simulink model "WEC_Model_SIMU"  (R2023b)
settings: Solver=ode4  StartTime=0.0  StopTime=20  FixedStep=50e-6  RelTol=1e-3
InitFcn:
  | load('Pgridwec.mat')
  | Lg=0.05;
  | rg=0.01;
  | kp_g=0.5*10.9;
  | ki_g=0.1*7.9e4;
  | Sbase=100e6;
  | Imax=1.5;
  | Vbase=132e3;
  | Ibase=5248.639;
libraries: slpidlib x2, spsPLL3phLib x1, spsabctodq0Lib x1, spsdq0toabcLib x1
settings Model: Creator=podde  LastModifiedBy=barajale

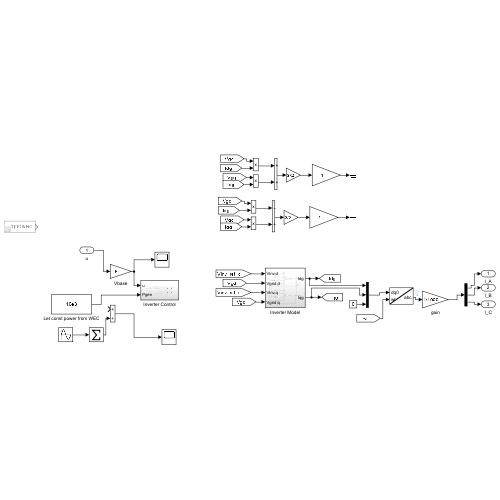
[thumbnail: Simulink's stored preview of the top-level diagram]
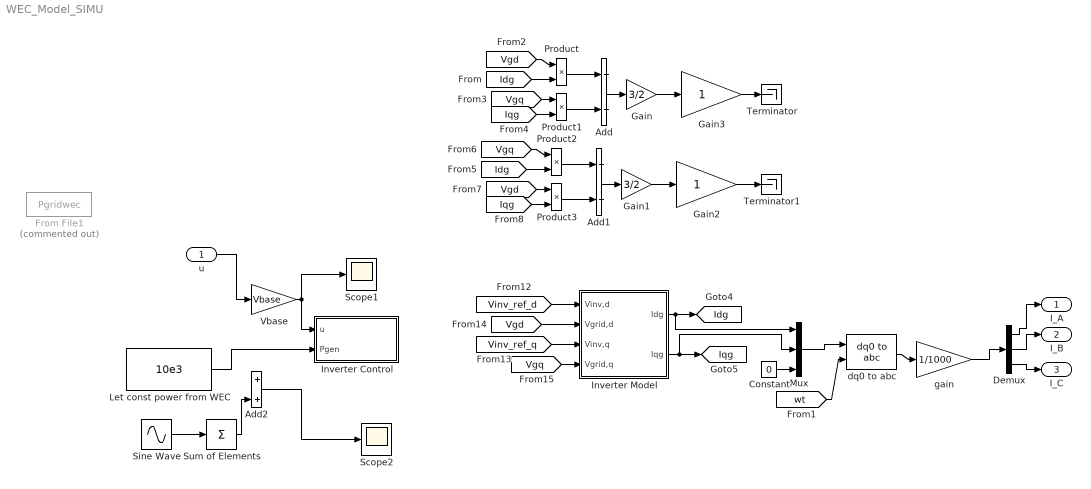
== system WEC_Model_SIMU ==
  u : Inport
  Add : Sum
  Add1 : Sum  Inputs=-+
  Add2 : Sum
  Constant : Constant  Value=0
  Demux : Demux  Outputs=3
  From File1 : FromFile  Commented=on  FileName=Pgridwec  SampleTime=0
  Gain : Gain  Gain=3/2
  Gain1 : Gain  Gain=3/2
  Gain2 : Gain
  Gain3 : Gain
  Inverter Control : Subsystem
  Inverter Model : Subsystem
  Let const power from WEC : Constant  Value=10e3
  Mux : Mux  Inputs=3
  Product{,1..3} (4 alike) : Product
  Scope1 : Scope
  Scope2 : Scope
  Sine Wave : Sin  Amplitude=0  Frequency=[2*pi/3 2*pi/5 2*pi/7]  Phase=[0,-2*pi/3, 2*pi/3]  SampleTime=0
  Sum of Elements : Sum  Inputs=+
  Terminator : Terminator
  Terminator1 : Terminator
  Vbase : Gain  Gain=Vbase
  dq0 to abc : spsdq0toabcLib/dq0 to abc  Alignment=90 degrees behind phase A axis
  gain : Gain  Gain=1/1000
  I_A : Outport
  I_B : Outport  Port=2
  I_C : Outport  Port=3
  tag scope: Idg=global, Iqg=global
  wires:
  Inverter Model/1(Idg) -> Mux/1, [Idg]
  Inverter Model/2(Iqg) -> Mux/2, [Iqg]
  [Vinv_ref_d] -> Inverter Model/1(Vinv,d)
  [Vgd] -> Inverter Model/2(Vgrid,d)
  [Vinv_ref_q] -> Inverter Model/3(Vinv,q)
  [Vgq] -> Inverter Model/4(Vgrid,q)
  Constant/1 -> Mux/3
  Mux/1 -> dq0 to abc/1
  [wt] -> dq0 to abc/2
  Demux/2 -> I_B/1
  Demux/3 -> I_C/1
  [Vgd] -> Product/1
  [Idg] -> Product/2
  [Vgq] -> Product1/1
  [Iqg] -> Product1/2
  Product/1 -> Add/1
  Product1/1 -> Add/2
  Add/1 -> Gain/1
  Product3/1 -> Add1/2
  [Vgq] -> Product2/1
  [Idg] -> Product2/2
  [Vgd] -> Product3/1
  Product2/1 -> Add1/1
  Add1/1 -> Gain1/1
  [Iqg] -> Product3/2
  Gain1/1 -> Gain2/1
  Gain2/1 -> Terminator1/1
  Gain/1 -> Gain3/1
  Gain3/1 -> Terminator/1
  Demux/1 -> I_A/1
  Vbase/1 -> Inverter Control/1(u), Scope1/1
  u/1 -> Vbase/1
  gain/1 -> Demux/1
  dq0 to abc/1 -> gain/1
  Sum of Elements/1 -> Add2/2
  Let const power from WEC/1 -> Inverter Control/2(Pgen)
  Add2/1 -> Scope2/1
  Sine Wave/1 -> Sum of Elements/1

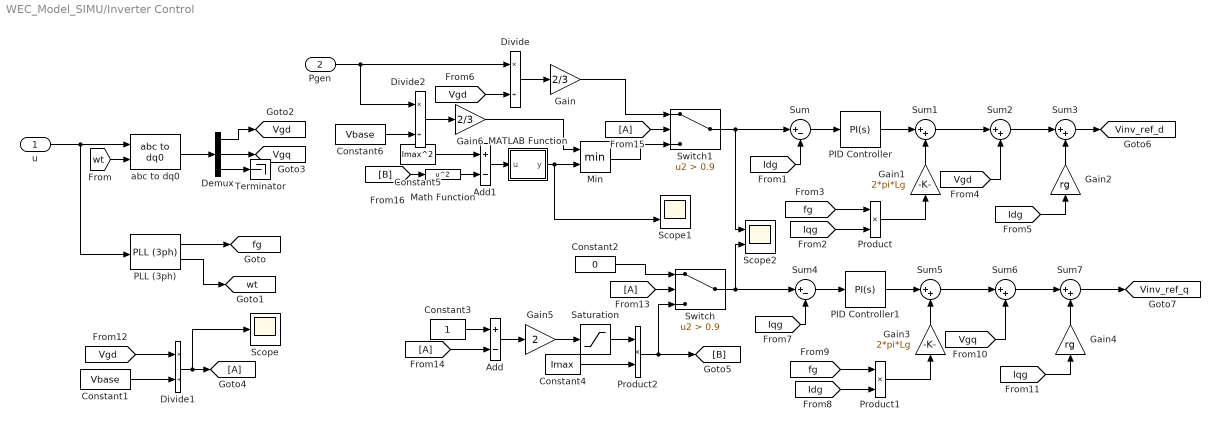
== system WEC_Model_SIMU/Inverter Control ==
  u : Inport
  Pgen : Inport  Port=2
  Add : Sum  Inputs=+-
  Add1 : Sum  Inputs=+-
  Constant1 : Constant  Value=Vbase
  Constant2 : Constant  Value=0
  Constant3 : Constant
  Constant4 : Constant  Value=Imax
  Constant5 : Constant  Value=Imax^2
  Constant6 : Constant  Value=Vbase
  Demux : Demux  Outputs=3
  Divide : Product  Inputs=*/
  Divide1 : Product  Inputs=*/
  Divide2 : Product  Inputs=*/
  From13 : From
  From14 : From
  From15 : From
  Gain : Gain  Gain=2/3
  Gain1 : Gain  Gain=2*pi*Lg
  Gain2 : Gain  Gain=rg
  Gain3 : Gain  Gain=2*pi*Lg
  Gain4 : Gain  Gain=rg
  Gain5 : Gain  Gain=2
  Gain6 : Gain  Gain=2/3
  Goto4 : Goto
  MATLAB Function : MATLAB Function  TreatAsAtomicUnit=on
  Math Function : Math  Operator=square
  Min : MinMax  Inputs=2
  PID Controller : slpidlib/PID Controller  Controller=PI  Form=Parallel  TimeDomain=Continuous-time  UseExternalTs=off  SampleTime=-1  IntegratorMethod=Forward Euler  FilterMethod=Forward Euler  ControllerParametersSource=internal  P=kp_g  I=ki_g  UseKiTs=off  D=0  N=100  UseFilter=on  TunerSelectOption=Transfer Function Based (PID Tuner App)  InitialConditionSource=internal  InitialConditionForIntegrator=0  InitialConditionForFilter=0  DifferentiatorICPrevScaledInput=0  ExternalReset=none  TrackingMode=off  Kt=1  LimitOutput=off  SatLimitsSource=internal  UpperSaturationLimit=inf  LowerSaturationLimit=-inf  LinearizeAsGain=on  AntiWindupMode=none  Kb=1  LimitIntegrator=off  UpperIntegratorSaturationLimit=inf  LowerIntegratorSaturationLimit=-inf  POutMin=[]  POutMax=[]  IOutMin=[]  IOutMax=[]  DOutMin=[]  DOutMax=[]  NOutMin=[]  NOutMax=[]  SumOutMin=[]  SumOutMax=[]  SaturationOutMin=[]  SaturationOutMax=[]  PParamMin=[]  PParamMax=[]  IParamMin=[]  IParamMax=[]  DParamMin=[]  DParamMax=[]  NParamMin=[]  NParamMax=[]  KbParamMin=[]  KbParamMax=[]  KtParamMin=[]  KtParamMax=[]  KbOutMin=[]  KbOutMax=[]  KtOutMin=[]  KtOutMax=[]  IntegratorOutMin=[]  IntegratorOutMax=[]  FilterOutMin=[]  FilterOutMax=[]  SumI1OutMin=[]  SumI1OutMax=[]  SumI2OutMin=[]  SumI2OutMax=[]  SumI3OutMin=[]  SumI3OutMax=[]  SumI4OutMin=[]  SumI4OutMax=[]  SumDOutMin=[]  SumDOutMax=[]  DifferentiatorOutMin=[]  DifferentiatorOutMax=[]  FilterDiffOutCoefMin=[]  FilterDiffOutCoefMax=[]  ReciprocalOutMin=[]  ReciprocalOutMax=[]  SumDenOutMin=[]  SumDenOutMax=[]  SumNumOutMin=[]  SumNumOutMax=[]  DivideOutMin=[]  DivideOutMax=[]  UdiffTsProdOutMin=[]  UdiffTsProdOutMax=[]  NTsProdOutMin=[]  NTsProdOutMax=[]  UintegralTsProdOutMin=[]  UintegralTsProdOutMax=[]  UngainTsProdOutMin=[]  UngainTsProdOutMax=[]  ClampingZeroOutDataTypeStr=Inherit: Inherit via back propagation  ClampingZeroOutMin=[]  ClampingZeroOutMax=[]  FilterDenConstantOutDataTypeStr=Inherit: Inherit via back propagation  FilterDenConstantOutMin=[]  FilterDenConstantOutMax=[]  PCopyOutDataTypeStr=Inherit: Inherit via back propagation  PCopyOutMin=[]  PCopyOutMax=[]  NCopyOutDataTypeStr=Inherit: Inherit via back propagation  NCopyOutMin=[]  NCopyOutMax=[]  IntegratorContinuousStateAttributes=''  IntegratorStateMustResolveToSignalObject=off  IntegratorRTWStateStorageClass=Auto  FilterContinuousStateAttributes=''  FilterStateMustResolveToSignalObject=off  FilterRTWStateStorageClass=Auto  ParallelPVariant=InternalParameters  IdealPVariant=Disabled  IVariant=InternalParameters  DVariant=Disabled  IntegratorVariant=Continuous  SatVariant=Disabled  AWVariant=Passthrough  PCopyVariant=Disabled  TRVariant=Disabled  FdbkBlocksVariant=Forward  IdealPFdbkVariant=Disabled  SatFdbkVariant=Disabled  DerivativeFilterVariant=Disabled  NVariant=Disabled  NCopyVariant=Disabled_SignalSpec  FilterICVariant=Disabled  IntegratorICVariant=InternalICs  ExternalResetVariant=Disabled  TRSumVariant=Passthrough  SumFdbkVariant=Disabled  SumVariant=Sum_PI  TsampFilterVariant=InternalTs  TsampNgainVariant=Passthrough  TsampIntegralVariant=Disabled_SignalSpec  ExternalSaturationOutDataTypeStr=Inherit: Same as second input
  PID Controller1 : slpidlib/PID Controller  Controller=PI  Form=Parallel  TimeDomain=Continuous-time  UseExternalTs=off  SampleTime=-1  IntegratorMethod=Forward Euler  FilterMethod=Forward Euler  ControllerParametersSource=internal  P=kp_g  I=ki_g  UseKiTs=off  D=0  N=100  UseFilter=on  TunerSelectOption=Transfer Function Based (PID Tuner App)  InitialConditionSource=internal  InitialConditionForIntegrator=0  InitialConditionForFilter=0  DifferentiatorICPrevScaledInput=0  ExternalReset=none  TrackingMode=off  Kt=1  LimitOutput=off  SatLimitsSource=internal  UpperSaturationLimit=inf  LowerSaturationLimit=-inf  LinearizeAsGain=on  AntiWindupMode=none  Kb=1  LimitIntegrator=off  UpperIntegratorSaturationLimit=inf  LowerIntegratorSaturationLimit=-inf  POutMin=[]  POutMax=[]  IOutMin=[]  IOutMax=[]  DOutMin=[]  DOutMax=[]  NOutMin=[]  NOutMax=[]  SumOutMin=[]  SumOutMax=[]  SaturationOutMin=[]  SaturationOutMax=[]  PParamMin=[]  PParamMax=[]  IParamMin=[]  IParamMax=[]  DParamMin=[]  DParamMax=[]  NParamMin=[]  NParamMax=[]  KbParamMin=[]  KbParamMax=[]  KtParamMin=[]  KtParamMax=[]  KbOutMin=[]  KbOutMax=[]  KtOutMin=[]  KtOutMax=[]  IntegratorOutMin=[]  IntegratorOutMax=[]  FilterOutMin=[]  FilterOutMax=[]  SumI1OutMin=[]  SumI1OutMax=[]  SumI2OutMin=[]  SumI2OutMax=[]  SumI3OutMin=[]  SumI3OutMax=[]  SumI4OutMin=[]  SumI4OutMax=[]  SumDOutMin=[]  SumDOutMax=[]  DifferentiatorOutMin=[]  DifferentiatorOutMax=[]  FilterDiffOutCoefMin=[]  FilterDiffOutCoefMax=[]  ReciprocalOutMin=[]  ReciprocalOutMax=[]  SumDenOutMin=[]  SumDenOutMax=[]  SumNumOutMin=[]  SumNumOutMax=[]  DivideOutMin=[]  DivideOutMax=[]  UdiffTsProdOutMin=[]  UdiffTsProdOutMax=[]  NTsProdOutMin=[]  NTsProdOutMax=[]  UintegralTsProdOutMin=[]  UintegralTsProdOutMax=[]  UngainTsProdOutMin=[]  UngainTsProdOutMax=[]  ClampingZeroOutDataTypeStr=Inherit: Inherit via back propagation  ClampingZeroOutMin=[]  ClampingZeroOutMax=[]  FilterDenConstantOutDataTypeStr=Inherit: Inherit via back propagation  FilterDenConstantOutMin=[]  FilterDenConstantOutMax=[]  PCopyOutDataTypeStr=Inherit: Inherit via back propagation  PCopyOutMin=[]  PCopyOutMax=[]  NCopyOutDataTypeStr=Inherit: Inherit via back propagation  NCopyOutMin=[]  NCopyOutMax=[]  IntegratorContinuousStateAttributes=''  IntegratorStateMustResolveToSignalObject=off  IntegratorRTWStateStorageClass=Auto  FilterContinuousStateAttributes=''  FilterStateMustResolveToSignalObject=off  FilterRTWStateStorageClass=Auto  ParallelPVariant=InternalParameters  IdealPVariant=Disabled  IVariant=InternalParameters  DVariant=Disabled  IntegratorVariant=Continuous  SatVariant=Disabled  AWVariant=Passthrough  PCopyVariant=Disabled  TRVariant=Disabled  FdbkBlocksVariant=Forward  IdealPFdbkVariant=Disabled  SatFdbkVariant=Disabled  DerivativeFilterVariant=Disabled  NVariant=Disabled  NCopyVariant=Disabled_SignalSpec  FilterICVariant=Disabled  IntegratorICVariant=InternalICs  ExternalResetVariant=Disabled  TRSumVariant=Passthrough  SumFdbkVariant=Disabled  SumVariant=Sum_PI  TsampFilterVariant=InternalTs  TsampNgainVariant=Passthrough  TsampIntegralVariant=Disabled_SignalSpec  ExternalSaturationOutDataTypeStr=Inherit: Same as second input
  PLL (3ph) : spsPLL3phLib/PLL (3ph)  Fmin=45  Par_Init=[0, 60]  ParK=[180, 3200, 1]  TcD=1e-4  MaxRateChangeFreq=12  FilterCutOffFreq=25  Ts=0  AGC=on
  Product : Product
  Product1 : Product
  Product2 : Product
  Saturation : Saturate  UpperLimit=1  LowerLimit=0
  Scope : Scope
  Scope1 : Scope  NumInputPorts=2
  Scope2 : Scope  NumInputPorts=2
  Sum : Sum  Inputs=|+-
  Sum{1..3,5..7} (6 alike) : Sum  Inputs=|++
  Sum4 : Sum  Inputs=|+-
  Switch : Switch  Criteria=u2 > Threshold  Threshold=0.9  SaturateOnIntegerOverflow=off  InputSameDT=off
  Switch1 : Switch  Criteria=u2 > Threshold  Threshold=0.9  SaturateOnIntegerOverflow=off  InputSameDT=off
  Terminator : Terminator
  abc to dq0 : spsabctodq0Lib/abc to dq0  Alignment=90 degrees behind phase A axis
  tag scope: Vgd=global, Vgq=global, Vinv_ref_d=global, Vinv_ref_q=global, fg=global, wt=global
  wires:
  [Idg] -> Product1/2
  abc to dq0/1 -> Demux/1
  [Idg] -> Gain2/1
  Sum4/1 -> PID Controller1/1
  [Iqg] -> Sum4/2
  Gain4/1 -> Sum7/2
  [Iqg] -> Gain4/1
  Divide/1 -> Gain/1
  PID Controller1/1 -> Sum5/1
  Sum/1 -> PID Controller/1
  Sum5/1 -> Sum6/1
  Gain3/1 -> Sum5/2
  [Vgq] -> Sum6/2
  Sum6/1 -> Sum7/1
  PLL (3ph)/2 -> [wt]
  Gain1/1 -> Sum1/2
  [fg] -> Product1/1
  Sum2/1 -> Sum3/1
  Product1/1 -> Gain3/1
  Sum3/1 -> [Vinv_ref_d]
  u/1 -> PLL (3ph)/1, abc to dq0/1
  Switch/1 -> Scope2/2, Sum4/1
  PLL (3ph)/1 -> [fg]
  Demux/3 -> Terminator/1
  [Idg] -> Sum/2
  Demux/2 -> [Vgq]
  Sum1/1 -> Sum2/1
  Demux/1 -> [Vgd]
  [wt] -> abc to dq0/2
  Gain2/1 -> Sum3/2
  PID Controller/1 -> Sum1/1
  [fg] -> Product/1
  Product/1 -> Gain1/1
  [Vgd] -> Divide/2
  [Vgd] -> Sum2/2
  [Iqg] -> Product/2
  [Vgd] -> Divide1/1
  Constant1/1 -> Divide1/2
  Divide1/1 -> Scope/1, Goto4/1
  From13/1 -> Switch/2
  Constant2/1 -> Switch/1
  Add/1 -> Gain5/1
  Constant3/1 -> Add/1
  From14/1 -> Add/2
  Gain5/1 -> Saturation/1
  Saturation/1 -> Product2/1
  Constant4/1 -> Product2/2
  Product2/1 -> Switch/3, [B]
  From15/1 -> Switch1/2
  Constant5/1 -> Add1/1
  [B] -> Math Function/1
  Math Function/1 -> Add1/2
  Add1/1 -> MATLAB Function/1(u)
  Switch1/1 -> Sum/1, Scope2/1
  Min/1 -> Switch1/3
  MATLAB Function/1(y) -> Scope1/2, Min/2
  Gain/1 -> Switch1/1
  Pgen/1 -> Divide2/1, Divide/1
  Divide2/1 -> Gain6/1
  Constant6/1 -> Divide2/2
  Gain6/1 -> Min/1
  Sum7/1 -> [Vinv_ref_q]

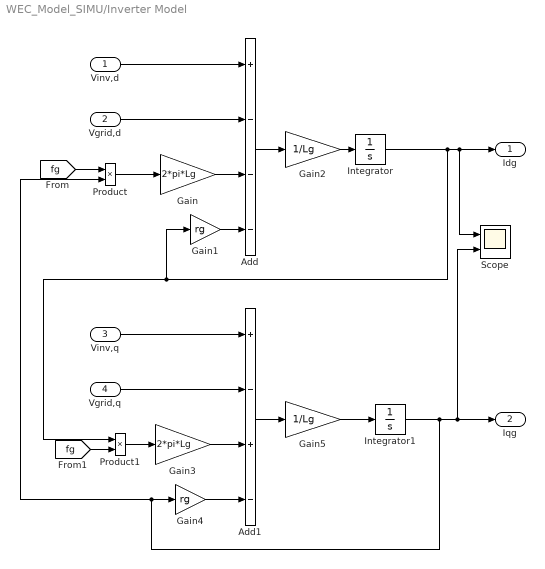
== system WEC_Model_SIMU/Inverter Model ==
  Vinv,d : Inport
  Vgrid,d : Inport  Port=2
  Vinv,q : Inport  Port=3
  Vgrid,q : Inport  Port=4
  Add : Sum  Inputs=+---
  Add1 : Sum  Inputs=+-+-
  Gain : Gain  Gain=2*pi*Lg
  Gain1 : Gain  Gain=rg
  Gain2 : Gain  Gain=1/Lg
  Gain3 : Gain  Gain=2*pi*Lg
  Gain4 : Gain  Gain=rg
  Gain5 : Gain  Gain=1/Lg
  Integrator : Integrator
  Integrator1 : Integrator  InitialCondition=0.015
  Product : Product
  Product1 : Product
  Scope : Scope  NumInputPorts=2
  Idg : Outport
  Iqg : Outport  Port=2
  wires:
  Gain2/1 -> Integrator/1
  Gain1/1 -> Add/4
  Integrator/1 -> Scope/1, Idg/1, Product1/1, Gain1/1
  Gain3/1 -> Add1/3
  Vgrid,d/1 -> Add/2
  Add1/1 -> Gain5/1
  Integrator1/1 -> Scope/2, Iqg/1, Product/2, Gain4/1
  Add/1 -> Gain2/1
  Product/1 -> Gain/1
  Gain5/1 -> Integrator1/1
  Vgrid,q/1 -> Add1/2
  Vinv,d/1 -> Add/1
  Product1/1 -> Gain3/1
  [fg] -> Product1/2
  Gain4/1 -> Add1/4
  [fg] -> Product/1
  Gain/1 -> Add/3
  Vinv,q/1 -> Add1/1

== matlab function WEC_Model_SIMU/Inverter Control/MATLAB Function ==
  data: u input; y output
function y = fcn(u)

y = sqrt(u);
